simulink model "three_phase_npc_inverter"  (Simulink 7.3)
settings: Solver=ode45  StartTime=0.0  StopTime=0.1  RelTol=1e-3
InitFcn:
  | % Processor selection for I/O assignment
  | % The chosen Target in the Coder Options window must match the selected MCU.
  | % Set the variable 'type_evm' to the following strings to choose a specific target:
  | 
  |   type_evm = 'TI28379LP';     % TI28379D Delfino Launchpad
  | % type_evm = 'TI28379CC';  % TI28379D Delfino Controlcard
  | % type_evm = 'TI28388D';    % TI28388D Controlcard
  | 
  | % Configure I/O based on processor
  | switch (type_evm)
  | 	case 'TI28379LP'
  | 	% Configuration for TI28379D Launchpad
  | 	% On the Plant side
  | 		AO_RTBox_Vdc = 11;
  | 		AO_RTBox_Vmid = 3;
  | 		AO_RTBox_Vg = [4 5 6];
  | 		AO_RTBox_Ig = [12 13 14];
  | 		AO_RTBox_Icap = [9 1 15];
  | 		PWMCAP_RTBox_Qu = [0 2 1 3];
  | 		PWMCAP_RTBox_Qv = [4 16 5 17];
  | 		PWMCAP_RTBox_Qw = [18 20 19 21];
  | 		DO_RTBox_Eno = 4;
  | 		DI_RTBox_Power = 23;
  | 
  | 	% On the MCU side
  | 		ADC_DSP_ADCA = [2 4 5 3 1];
  | 		ADC_DSP_ADC2_select = 2;
  | 		ADC_DSP_ADC2 = [2 4];
  | 		ADC_DSP_ADC3_select = 3;
  | 		ADC_DSP_ADC3 = [2 4 5 3];
  | 		PWM_DSP_PWM = 1:6;
  | 		DO_DSP_LED = 34;
  | 		DI_DSP_En = 24;
  | 		PWR_DSP_GPIO = 131;
  | 
  | 		SCI_DSP = [43, 42];
  | 		AO_Factor = 1;
  | 		AO_Vmax = 3.3;
  | 
  | 	case 'TI28379CC'
  | 	% Configuration for TI28379D Controlcard
  | 	% On the Plant side
  | 		AO_RTBox_Vdc = 11;
  | 		AO_RTBox_Vmid = 9;
  | 		AO_RTBox_Vg = [14 2 15];
  | 		AO_RTBox_Ig = [12 0 13];
  | 		AO_RTBox_Icap = [10 8 7];
  | 		PWMCAP_RTBox_Qu = [0 2 1 3];
  | 		PWMCAP_RTBox_Qv = [4 6 5 7];
  | 		PWMCAP_RTBox_Qw = [8 10 9 11];
  | 		DO_RTBox_Eno = 21;
  | 		DI_RTBox_Power = 14;
  | 
  | 		% On the MCU side
  | 		ADC_DSP_ADCA = [0 1 2 3 4];
  | 		ADC_DSP_ADC2_select = 4;
  | 		ADC_DSP_ADC2 = [0 1];
  | 		ADC_DSP_ADC3_select = 2;
  | 		ADC_DSP_ADC3 = [0 1 2 3];
  | 		PWM_DSP_PWM = 1:6;
  | 		DO_DSP_LED = 34;
  | 		DI_DSP_En = 40;
  | 		PWR_DSP_GPIO = 39;
  | 
  | 		SCI_DSP = [28, 29];
  | 		AO_Factor = 1.54; % breakout board scaling 6.8k/4.42k
  | 		AO_Vmax = 5.0;
  | 
  | 	case 'TI28388D'
  | 	% Configuration for TI28388D Controlcard
  | 	% On the Plant side
  | 		AO_RTBox_Vdc = 11;
  | 		AO_RTBox_Vmid = 9;
  | 		AO_RTBox_Vg = [14 2 15];
  | 		AO_RTBox_Ig = [12 0 13];
  | 		AO_RTBox_Icap = [10 8 7];
  | 		PWMCAP_RTBox_Qu = [0 2 1 3];
  | 		PWMCAP_RTBox_Qv = [4 6 5 7];
  | 		PWMCAP_RTBox_Qw = [8 10 9 11];
  | 		DO_RTBox_Eno = 21;
  | 		DI_RTBox_Power = 14;
  | 
  | 		% On the MCU side
  | 		ADC_DSP_ADCA = [0 1 2 3 4];
  | 		ADC_DSP_ADC2_select = 4;
  | 		ADC_DSP_ADC2 = [0 1];
  | 		ADC_DSP_ADC3_select = 2;
  | 		ADC_DSP_ADC3 = [0 1 2 3];
  | 		PWM_DSP_PWM = 1:6;
  | 		DO_DSP_LED = 34;
  | 		DI_DSP_En = 40;
  | 		PWR_DSP_GPIO = 39;
  | 
  | 		SCI_DSP = [28, 29];
  | 		AO_Factor = 1.54; % breakout board scaling 6.8k/4.42k
  | 		AO_Vmax = 5.0;
  | 
  | 	otherwise
  | 	error('Unknown evaluation module selection, please choose either ''TI28379LP'', ''TI28379CC'' or ''TI28388D''.')
  | end
  | 
  | 
  | %% Converter
  | fsw = 20e3; 					% switching frequency in Hz
  | 
  | %% Grid parameters
  | Vgrid_rms = 230;  				% Grid RMS volatge in V
  | Vll = sqrt(3)*Vgrid_rms;
  | Fgrid = 50;
  | Pn = 5e4; 					% nominal output 50 kW
  | 
  | %% HIL simulation
  | Ts_plant = 7e-6;  			          % discretization step size of the plant in s
  | Ts_ctrl = 1/fsw;  				% discretization step size of the controller in s
  | 
  | Adc_full = 3.0;
  | 
  | % DC voltage sensing
  | Vdcm.K = Adc_full / 1000; 		% full scale = 1000 V
  | 
  | % AC voltage sensing gain and offset
  | Vacm.K = Adc_full / (2*1000);               % full scale = 2x1000 V
  | Vacm.O = Adc_full / 2.0;
  | 
  | % AC current sensing gain and offset
  | Iacm.K = Adc_full / (2*375); 	           % full scale = 2x375 A
  | Iacm.O = Adc_full / 2.0;
  | 
  | % Filter capacitor current sensing gain and offset
  | Icapm.K = Adc_full / (2*200);                % full scale = 2x200 A
  | Icapm.O = Adc_full / 2.0;
  | 
  | %% LCL filter design
  | Zb = Vll^2/Pn;
  | Cb = 1/(2*pi*Fgrid*Zb);
  | Lb = Zb/(2*pi*Fgrid);
  | Cf = 0.05*Cb; 				 % filter capacitance
  | Ldc = 0.1*Lb;
  | Lc = 0.5*Ldc; 				 % first stage filter inductance
  | Lg = 0.5*Ldc; 				 % second stage filter inductance
  | Leq = Lc*Lg/(Lc+Lg); 			 % equivalent inductance for resonance (Lc/Lg)
  | Fres = 1/2/pi/sqrt(Leq*Cf); 	           % LCL resonant frequency
  | RD = 1/3/(2*pi*Fres*Cf); 		           % passive damping resistor
  | L_f = Lc + Lg; 				 % equivalent L for dq model
  | R = 0.05; 					 % fiter inductor resistance
  | R_f = 2*R; 					 % equivalent R for dq model
  | 
  | %% Current PI controller design
  | Id_ref = Pn/3/Vgrid_rms*sqrt(2);
  | Tn = L_f/R_f;
  | Ti = 10*(1/R_f)*Ts_ctrl;
  | Kp = Tn/Ti;
  | Ki = 1/Ti;
  | Kbc = Ki/Kp;
undefined symbols (not defined in the file): plecs
settings Model: Creator=kris  LastModifiedBy=manaswini  ExtModeTrigMode=oneshot  ExtModeArmWhenConnect=off  ExtModeAutoUpdateStatusClock=off
settings DataIOCC: LimitDataPoints=off  ReturnWorkspaceOutputs=off  SignalLoggingName=sigsOut
settings OptimizationCC: BooleanDataType=off  ExpressionDepthLimit=128  InitFltsAndDblsToZero=on
settings DebuggingCC: SaveWithParameterizedLinksMsg=none  SignalResolutionControl=TryResolveAllWithWarning  SolverPrmCheckMsg=none  MultiTaskDSMMsg=warning  MultiTaskCondExecSysMsg=none  FcnCallInpInsideContextMsg=Enable All  StrictBusMsg=ErrorLevel1
settings HardwareCC: TargetHWDeviceType=32-bit Generic  TargetUnknown=on  ProdEqTarget=off
settings RTWCC: IncludeERTFirstTime=on
settings CodeAppCC: CustomSymbolStrType=$N$R$M_T
settings GRTTargetCC: TargetFcnLib=ansi_tfl_tmw.mat  TargetFunctionLibrary=C89/C90 (ANSI)  ModelReferenceCompliant=off

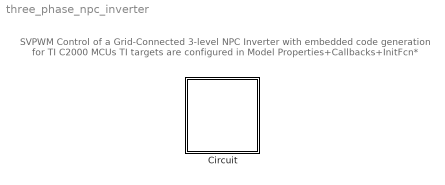
== system three_phase_npc_inverter ==
  note: SVPWM Control of a Grid-Connected 3-level NPC Inverter
      | with embedded code generation for TI C2000 MCUs
      | TI targets are configured in Model Properties+Callbacks+InitFcn*
  Circuit : Subsystem  LoadFcn=plecs('sl', 200);  InitFcn=plecs('sl', 214);  StartFcn=plecs('sl', 208);  StopFcn=plecs('sl', 209);  ClipboardFcn=plecs('sl', 212, 44);  mask(PlecsCircuit){PLECSData=<binary blob, 35408 chars, not shown>}
      mask prompts: PLECSData "PLECS Data (Do not delete or modify!)"
      mask help: Drag this block into a Simulink model to create a new electrical circuit.
      mask init:
      | % PLACE CUSTOM INITIALIZATIONS ABOVE
      | % DO NOT REMOVE
      | plecs('sl', 215);
      | % DO NOT REMOVE
      settings: CopyFcn=plecs('sl', 203);  DeleteFcn=plecs('sl', 205);  UndoDeleteFcn=plecs('sl', 206);  PreSaveFcn=plecs('sl', 211);  PostSaveFcn=plecs('sl', 201);  NameChangeFcn=plecs('sl', 210);  DestroyFcn=plecs('sl', 207);  PreCopyFcn=plecs('sl', 216);  OpenFcn=plecs('sl', 202);  ErrorFcn=plerrorfcn
      mask Display: disp('PLECS\nCircuit')

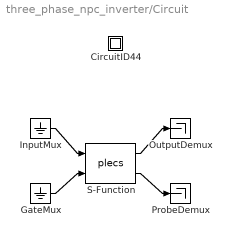
== system three_phase_npc_inverter/Circuit ==
  " CircuitID44 " : Subsystem
  " GateMux " : Ground
  " InputMux " : Ground
  " OutputDemux " : Terminator
  " ProbeDemux " : Terminator
  " S-Function " : S-Function  FunctionName=plecs  EnableBusSupport=off
  wires:
  " InputMux "/1 -> " S-Function "/1
  " GateMux "/1 -> " S-Function "/2
  " S-Function "/1 -> " OutputDemux "/1
  " S-Function "/2 -> " ProbeDemux "/1

== system three_phase_npc_inverter/Circuit/ CircuitID44  ==
